simulink model "EMPC_DUE"  (R2019a)
settings: Solver=FixedStepAuto  StartTime=0.0  StopTime=120  RelTol=1e-3  EnableMultiTasking=on
undefined symbols (not defined in the file): DiscIntNeverNeededParam, i0, sigbuilder_block, Ts, u0, y0
libraries: MagnetoLibrary x3
settings Model: SimulationMode=external  ExtModeTrigDuration=2  Creator=jakub  LastModifiedBy=jakub
settings OptimizationCC: EnhancedBackFolding=on  PassReuseOutputArgsAs=Individual arguments  MaxStackSize=64  OptimizeBlockOrder=speed  DifferentSizesBufferReuse=on  OptimizationCustomize=off
settings DebuggingCC: ParameterTunabilityLossMsg=error
settings HardwareCC: ProdBitPerPointer=32  ProdBitPerSizeT=32  ProdBitPerPtrDiffT=32  ProdLargestAtomicInteger=Long  ProdLargestAtomicFloat=Double  ProdWordSize=32  ProdHWDeviceType=ARM Compatible->ARM Cortex
settings SFSimCC: MATLABDynamicMemAlloc=off
settings RTWCC: SystemTargetFile=ert.tlc  HardwareBoard=Arduino Due  TLCOptions=-aInlineSetEventsForThisBaseRateFcn=TLC_FALSE -aSuppressMultiTaskScheduler=TLC_FALSE -aRateBasedStepFcn=1  TemplateMakefile=ert_default_tmf  GenerateReport=on  Toolchain=Arduino ARM  BuildConfiguration=Faster Runs  IncludeHyperlinkInReport=on  LaunchReport=on  GenerateTraceInfo=on  GenerateTraceReport=on  GenerateTraceReportSl=on  GenerateTraceReportSf=on  GenerateTraceReportEml=on
settings CodeAppCC: ForceParamTrailComments=on  IgnoreCustomStorageClasses=off  OperatorAnnotations=on  SimulinkDataObjDesc=on  SFDataObjDesc=on  InsertBlockDesc=on
settings ERTTargetCC: SupportContinuousTime=on  SupportNonInlinedSFcns=on  SupportVariableSizeSignals=on  ExtModeStaticAllocSize=24576

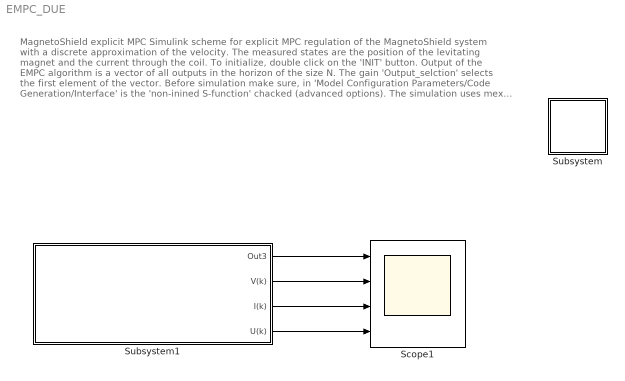
== system EMPC_DUE ==
  note: MagnetoShield explicit MPC
      | Simulink scheme for explicit MPC regulation of the MagnetoShield system with a discrete approximation of
      | the velocity. The measured states are the position of the levitating magnet and the current through the coil.
      | To initialize, double click on the 'INIT' button.
      | Output of the EMPC algorithm is a vector of all outputs in the horizon of the size N. The gain 'Output_selction'
      | selects the first element of the vector.
      |
      | Before simulation make sure, in 'Model Configuration Parameters/Code Generation/Interface' is the
      | 'non-inined S-function' chacked (advanced options).
      |
      | The simulation uses mex function 'ectrl_sfunc'. For the change of the default parameters, please use matlab
      | script 'MagnetoShield_Export_EMPC.m' and uncomment part 'Export for Simulink'. In the generate subfolder
      | 'empc' you can find a new mex function suitable for modified control problem with all needed souce files.
  Scope1 : Scope  NumInputPorts=4
  Subsystem : Subsystem
      settings: OpenFcn=|
      | clear; close all;clc;
      | cd(fileparts(which(gcs)));
      | load '../../../../../matlab/examples/MagnetoShield/MagnetoShield_Models_Greybox_SS';
      | 
      | 
      | Ts = 0.003;                      % Sampling
      mask Display: disp('INIT')
  Subsystem1 : Subsystem
  wires:
  Subsystem1/1(Out3) -> Scope1/1
  Subsystem1/2(V(k)) -> Scope1/2
  Subsystem1/3(I(k)) -> Scope1/3
  Subsystem1/4(U(k)) -> Scope1/4

== system EMPC_DUE/Subsystem ==

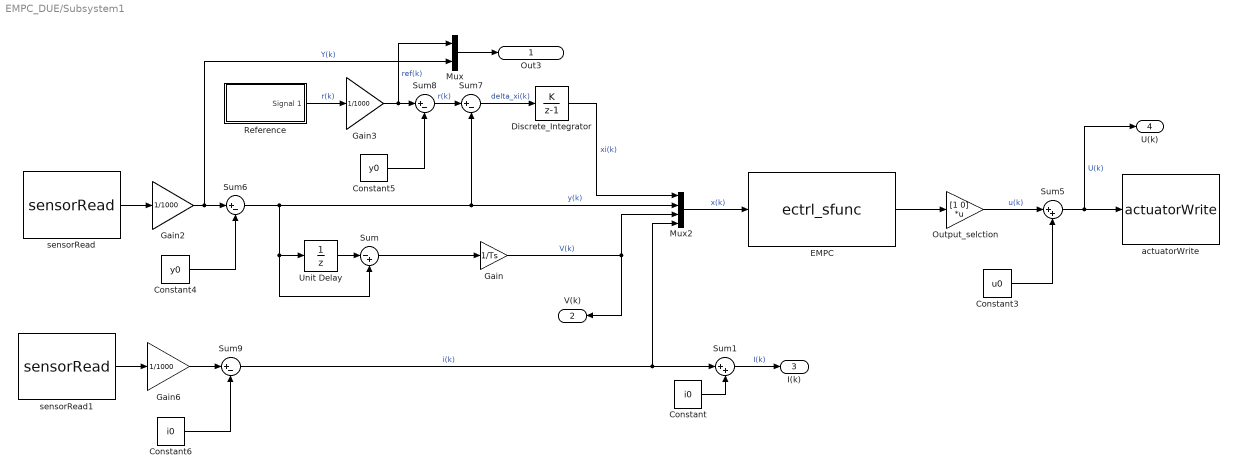
== system EMPC_DUE/Subsystem1 ==
  Constant : Constant  Value=i0
  Constant3 : Constant  Value=u0
  Constant4 : Constant  Value=y0
  Constant5 : Constant  Value=y0
  Constant6 : Constant  Value=i0
  Discrete_Integrator : DiscreteIntegrator  IntegratorMethod=Accumulation: Forward Euler  SampleTime=Ts  LimitOutput=on  UpperSaturationLimit=100  LowerSaturationLimit=-100  ICPrevOutput=DiscIntNeverNeededParam  ICPrevScaledInput=DiscIntNeverNeededParam
  EMPC : S-Function  FunctionName=ectrl_sfunc  SFunctionDeploymentMode=off  EnableBusSupport=off
  Gain : Gain  Gain=1/Ts
  Gain2 : Gain  Gain=1/1000
  Gain3 : Gain  Gain=1/1000
  Gain6 : Gain  Gain=1/1000
  Mux : Mux  Inputs=2
  Mux2 : Mux
  Output_selction : Gain  Gain=[1 0]  Multiplication=Matrix(K*u)
  Reference : Subsystem  Tag=STV Subsys  LoadFcn=sigbuilder_block('load');  StartFcn=sigbuilder_block('start');  StopFcn=sigbuilder_block('stop');  ClipboardFcn=sigbuilder_block('clipboard');  mask(Sigbuilder block){tuvar=[0:10]}
      mask help: Simulink:masks:SigbuilderBlock_MD
      mask init:
      | if ~strcmp(get_param(bdroot(gcbh),'SimulationStatus'),'stopped') tuvar = sigbuilder_block('maskInit'); end
      settings: CopyFcn=sigbuilder_block('copy');  DeleteFcn=sigbuilder_block('delete');  ModelCloseFcn=sigbuilder_block('modelClose');  PreSaveFcn=sigbuilder_block('preSave');  PauseFcn=sigbuilder_block('pause');  ContinueFcn=sigbuilder_block('continue');  NameChangeFcn=sigbuilder_block('namechange');  OpenFcn=sigbuilder_block('open',[61.8 52.2 1012.8 447.6 ]);  CloseFcn=sigbuilder_block('close');
      mask Display: plot(0, 0, 100, 100,[2, 2, 32, 32, 2], [68, 8, 8, 68, 68],[32, 2], [38, 38], [32, 19, 2],[53, 60, 44], [32, 17, 17, 2],[16, 16, 31, 31]);txt = getActiveGroup(gcbh);text(2, 100, txt,'verticalAlignment', 'top');
  Sum : Sum  Inputs=|-+
  Sum1 : Sum  Inputs=|++
  Sum5 : Sum  Inputs=|++
  Sum{6..9} (4 alike) : Sum  Inputs=|+-
  Unit Delay : UnitDelay  SampleTime=-1  HasFrameUpgradeWarning=on
  actuatorWrite : MagnetoLibrary/actuatorWrite  Board=DUE  Units=Volts
      settings: SourceProductName=AutomationShield
  sensorRead : MagnetoLibrary/sensorRead  board=DUE  sensor=Distance [mm]  sampling=Ts
      settings: SourceProductName=AutomationShield
  sensorRead1 : MagnetoLibrary/sensorRead  board=DUE  sensor=Current [mA]  sampling=Ts
      settings: SourceProductName=AutomationShield
  Out3 : Outport
  V(k) : Outport  Port=2
  I(k) : Outport  Port=3
  U(k) : Outport  Port=4
  wires:
  Sum5/1 -> U(k)/1, actuatorWrite/1  "U(k)"
  Constant6/1 -> Sum9/2
  Sum6/1 -> Mux2/2, Sum7/2, Unit Delay/1, Sum/2  "y(k)"
  Reference/1(Signal 1) -> Gain3/1  "r(k)"
  sensorRead/1 -> Gain2/1
  EMPC/1 -> Output_selction/1
  sensorRead1/1 -> Gain6/1
  Gain6/1 -> Sum9/1
  Constant3/1 -> Sum5/2
  Gain/1 -> Mux2/3, V(k)/1  "V(k)"
  Unit Delay/1 -> Sum/1
  Gain3/1 -> Mux/1, Sum8/1  "ref(k)"
  Constant5/1 -> Sum8/2
  Mux/1 -> Out3/1
  Gain2/1 -> Mux/2, Sum6/1  "Y(k)"
  Sum9/1 -> Mux2/4, Sum1/1  "i(k)"
  Sum/1 -> Gain/1
  Mux2/1 -> EMPC/1  "x(k)"
  Sum7/1 -> Discrete_Integrator/1  "delta_xi(k)"
  Discrete_Integrator/1 -> Mux2/1  "xi(k)"
  Output_selction/1 -> Sum5/1  "u(k)"
  Sum8/1 -> Sum7/1  "r(k)"
  Sum1/1 -> I(k)/1  "I(k)"
  Constant4/1 -> Sum6/2
  Constant/1 -> Sum1/2

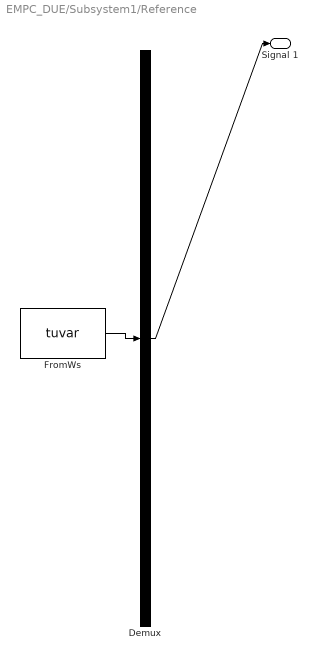
== system EMPC_DUE/Subsystem1/Reference ==
  Demux : Demux  Tag=STV Demux  Outputs=1
  FromWs : FromWorkspace  Tag=STV FromWs  VariableName=tuvar  SampleTime=0
      SigBuilderData=|
      | common.afterFinalStr = 'Extrapolate'
      | common.sampleTime = 0
      | dataSet.timeRange = [0 120]
      | dataSet.name = 'Group 1'
      | sbobj.Groups.Name = 'Group 1'
      | sbobj.Groups.Signals.Name = 'Signal 1'
      | sbobj.Groups.Signals.XData = [0 5 5 10 15 15 20 25 25 30 35 35 40 45 45 50 55 55 60 65 70 70 75 80 85 85 90 95 100 105 110 115 115 120]
      | sbobj.Groups.Signals.YData = [17 17 16.5 16.5 16.5 15.5 15.5 15.5 14.5 14.5 14.5 13.5 13.5 13.5 12.5 12.5 12.5 16 16 16 16 13.5 13.5 13.5 13.5 15 15 15 17 12 14.5 14.5 17 17]
      | sbobj.Groups.TimeRange = [0 120]
  Signal 1 : Outport  Tag=STV Outport
  wires:
  FromWs/1 -> Demux/1
  Demux/1 -> Signal 1/1
